simulink model "Intdmb"  (Simulink 8.1)
settings: Solver=VariableStepDiscrete  StartTime=0.0  StopTime=1000  RelTol=1e-3
undefined symbols (not defined in the file or in its folder): DiscIntNeverNeededParam
libraries: commchan3 x1, commdigbbndpm3 x1, commrandsrc2 x1, simulink_extras x1, dspsigops x1, commsink2 x1, simulink x1
settings Model: Creator=Gaurav  LastModifiedBy=Gaurav
settings DataIOCC: SignalLoggingSaveFormat=Dataset
settings OptimizationCC: ExpressionDepthLimit=128
settings DebuggingCC: FcnCallInpInsideContextMsg=EnableAllAsError
settings GRTTargetCC: CombineOutputUpdateFcns=on  GRTInterface=off

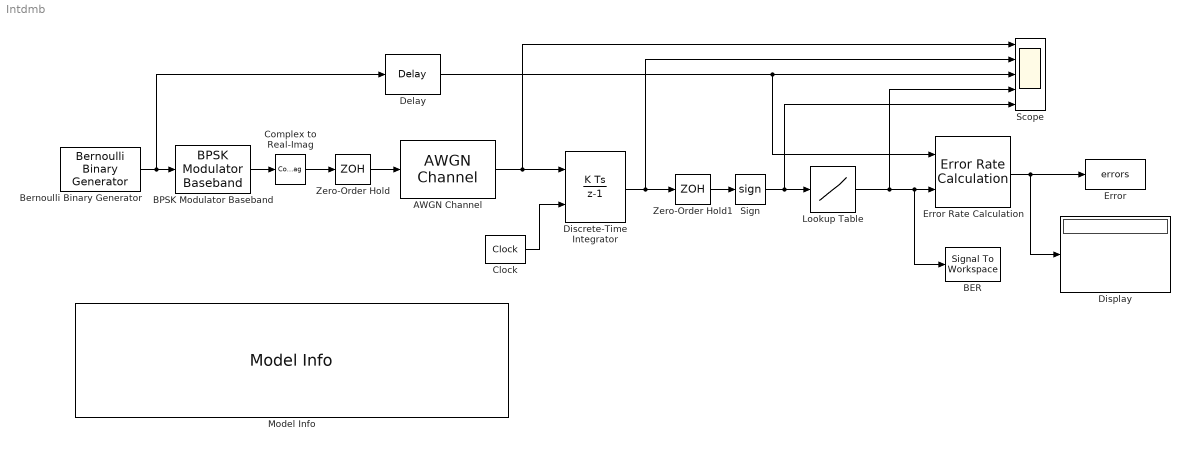
== system Intdmb ==
  AWGN Channel : commchan3/AWGN Channel  InputProcessing=Inherited (this choice will be removed - see release notes)  seed=69  noiseMode="Signal to noise ratio  (Eb/No)"  EbNodB=10  EsNodB=10  SNRdB=10  bitsPerSym=1  Ps=1  Tsym=1  variance=1
  BER : SignalToWorkspace  VariableName=BER
      settings: CopyFcn=dspblkcopystw(gcbh);
  BPSK Modulator Baseband : commdigbbndpm3/BPSK Modulator Baseband  Ph=0  outDtype=double  outWordLen=16  outUDDataType=sfix(16)  outFracLenMode=Best precision  outFracLen=15
  Bernoulli Binary Generator : commrandsrc2/Bernoulli Binary Generator  P=0.5  seed=61  Ts=1  frameBased=off  sampPerFrame=1  orient=off  outDataType=double
  Clock : simulink_extras/Flip Flops/Clock  period=1.000001
  Complex to Real-Imag : ComplexToRealImag  Output=Real
  Delay : dspsigops/Delay  InputProcessing=Columns as channels (frame based)  dly_unit=Samples  delay=1  ic_detail=off  dif_ic_for_ch=off  dif_ic_for_dly=off  ic=0  reset_popup=None
  Discrete-Time Integrator : DiscreteIntegrator  ExternalReset=rising  SampleTime=1/20  ICPrevOutput=DiscIntNeverNeededParam  ICPrevScaledInput=DiscIntNeverNeededParam
  Display : Display
  Error : ToWorkspace  VariableName=errors  SampleTime=-1
      settings: MaxDataPoints=1
  Error Rate Calculation : commsink2/Error Rate Calculation  N=0  st_delay=1  cp_mode=Entire frame  subframe=[]  PMode=Port  WsName=BER  RsMode2=off  stop=off  numErr=100  maxBits=1e6
  Lookup Table : Lookup  InputValues=[-1,1]  Table=[1,0]
  Model Info : simulink/Model-Wide Utilities/Model Info  InitialBlockCM=None  BlockCM=None  Frame=on  DisplayStringWithTags=|  HorizontalTextAlignment=Center  LeftAlignmentValue=0.5  SourceBlockDiagram=Intdmb  TagMaxNumber=20
      | %<Created>
      | Gaurav Sharma
      | %<ModifiedBy>
      | %<ModifiedDate>
      | BPSK BER in AWGN Using Integrater
      | The model is Run from Bpsk_Integrate_dumb.m file in the folder to generate BER curve
      | %<LastModifiedBy>
      | %<LastModificationDate>
  Scope : Scope  NumInputPorts=5
      settings: YMin=-3~-2~-2~-2~-2  YMax=3~2~2~2~2
  Sign : Signum
  Zero-Order Hold : ZeroOrderHold  SampleTime=0.1
  Zero-Order Hold1 : ZeroOrderHold
  wires:
  Lookup Table/1 -> BER/1, Error Rate Calculation/2, Scope/4
  Delay/1 -> Error Rate Calculation/1, Scope/3
  Clock/1 -> Discrete-Time Integrator/2
  Discrete-Time Integrator/1 -> Zero-Order Hold1/1, Scope/2
  Zero-Order Hold/1 -> AWGN Channel/1
  AWGN Channel/1 -> Discrete-Time Integrator/1, Scope/1
  Error Rate Calculation/1 -> Error/1, Display/1
  Sign/1 -> Scope/5, Lookup Table/1
  Zero-Order Hold1/1 -> Sign/1
  Bernoulli Binary Generator/1 -> BPSK Modulator Baseband/1, Delay/1
  BPSK Modulator Baseband/1 -> Complex to Real-Imag/1
  Complex to Real-Imag/1 -> Zero-Order Hold/1
